simulink model "rec_i2s"  (R2023b)
settings: Solver=VariableStepAuto  StartTime=0.0  StopTime=10  RelTol=1e-3
values from neighbouring files (symbols this model uses):
  cnt1_LRCLK = 511    [DATA_GEN.m]
  cnt2_SCLK = 7    [DATA_GEN.m]
libraries: hdlsllib x3, eeGeneralControl x1
settings Model: Creator=31651  LastModifiedBy=31651
settings OptimizationCC: BlockReduction=off  ConditionallyExecuteInputs=off

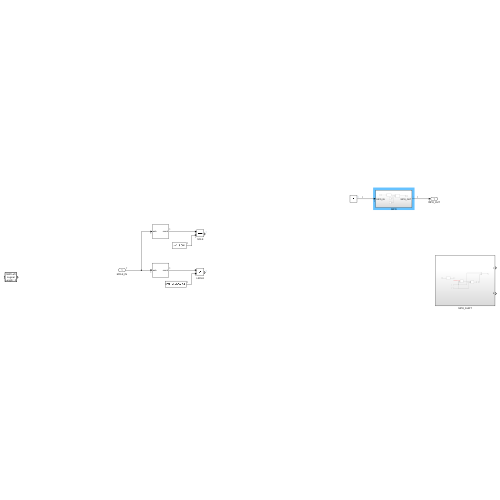
[thumbnail: Simulink's stored preview of the top-level diagram]
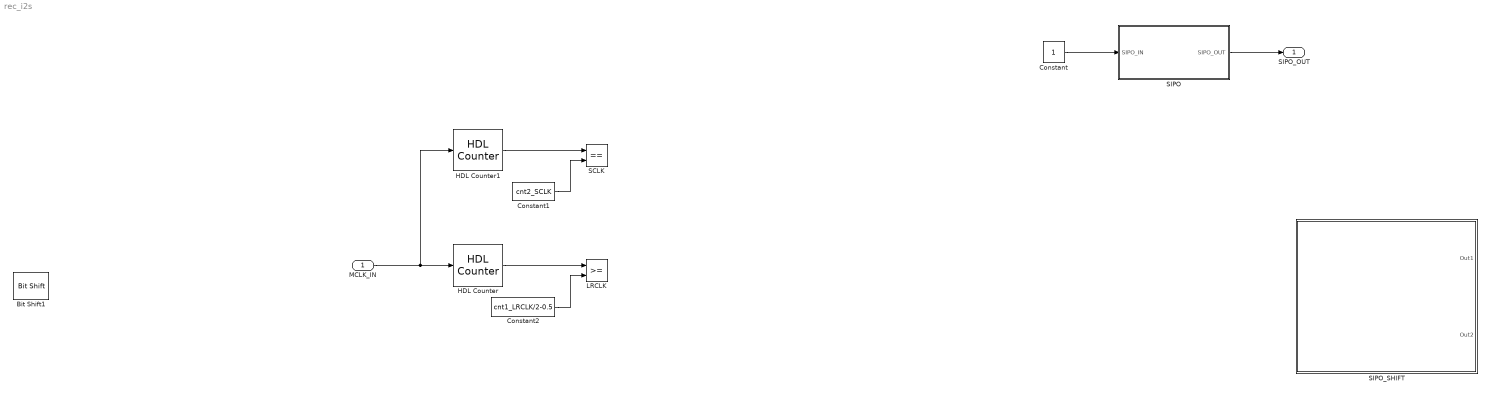
== system rec_i2s ==
  MCLK_IN : Inport
  Bit Shift1 : hdlsllib/Logic and Bit Operations/Bit Shift  mode=Shift Left Logical  N=0
  Constant : Constant  OutDataTypeStr=boolean  SampleTime=1
  Constant1 : Constant  Value=cnt2_SCLK  OutDataTypeStr=uint16
  Constant2 : Constant  Value=cnt1_LRCLK/2-0.5  OutDataTypeStr=uint16
  HDL Counter : hdlsllib/Sources/HDL Counter  CountType=Count limited  CountInit=0  CountStep=1  CountMax=cnt1_LRCLK  CountFromType=Initial value  CountFrom=0  CountResetPort=off  CountLoadPort=off  CountEnbPort=on  CountDirPort=off  CountHitOutputPort=off  CountDataType=Unsigned  CountWordLen=16  CountFracLen=0  CountSampTime=1
  HDL Counter1 : hdlsllib/Sources/HDL Counter  CountType=Count limited  CountInit=0  CountStep=1  CountMax=cnt2_SCLK  CountFromType=Initial value  CountFrom=0  CountResetPort=off  CountLoadPort=off  CountEnbPort=on  CountDirPort=off  CountHitOutputPort=off  CountDataType=Unsigned  CountWordLen=16  CountFracLen=0  CountSampTime=1
  LRCLK : RelationalOperator  OutDataTypeStr=boolean  InputSameDT=off
  SCLK : RelationalOperator  Operator===  OutDataTypeStr=boolean  InputSameDT=off
  SIPO : Subsystem
  SIPO_SHIFT : Subsystem
  SIPO_OUT : Outport  VectorParamsAs1DForOutWhenUnconnected=off
  wires:
  Constant1/1 -> SCLK/2
  HDL Counter1/1 -> SCLK/1
  Constant2/1 -> LRCLK/2
  MCLK_IN/1 -> HDL Counter/1, HDL Counter1/1
  HDL Counter/1 -> LRCLK/1
  Constant/1 -> SIPO/1(SIPO_IN)
  SIPO/1(SIPO_OUT) -> SIPO_OUT/1

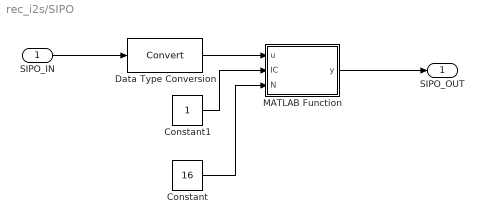
== system rec_i2s/SIPO ==
  SIPO_IN : Inport
  Constant : Constant  Value=16  SampleTime=1
  Constant1 : Constant  SampleTime=1
  Data Type Conversion : DataTypeConversion  SaturateOnIntegerOverflow=off  RndMeth=Floor
  MATLAB Function : MATLAB Function  TreatAsAtomicUnit=on
  SIPO_OUT : Outport  VectorParamsAs1DForOutWhenUnconnected=off
  wires:
  Data Type Conversion/1 -> MATLAB Function/1(u)
  MATLAB Function/1(y) -> SIPO_OUT/1
  SIPO_IN/1 -> Data Type Conversion/1
  Constant/1 -> MATLAB Function/3(N)
  Constant1/1 -> MATLAB Function/2(IC)

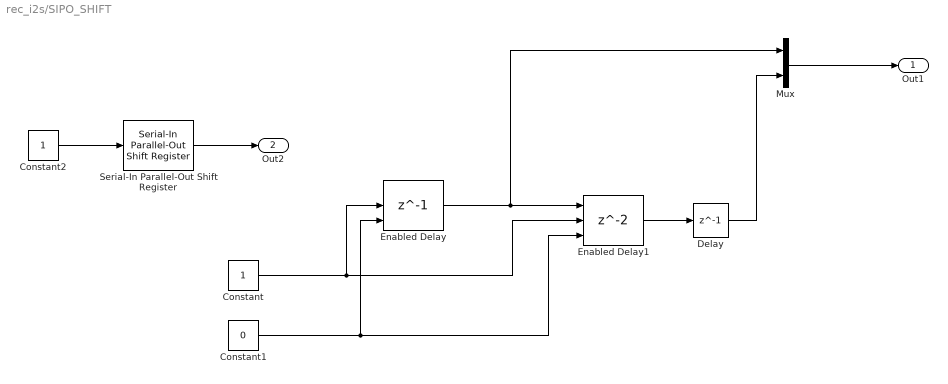
== system rec_i2s/SIPO_SHIFT ==
  Constant : Constant  OutDataTypeStr=boolean  SampleTime=1
  Constant1 : Constant  Value=0  OutDataTypeStr=boolean  SampleTime=1
  Constant2 : Constant  OutDataTypeStr=boolean  SampleTime=1
  Delay : Delay  DelayLength=1  InitialCondition=0
  Enabled Delay : Delay  DelayLength=1  ExternalReset=Level  ShowEnablePort=on
      settings: InputPortMap=u0,e6,r5
  Enabled Delay1 : Delay  ExternalReset=Level  ShowEnablePort=on
      settings: InputPortMap=u0,e6,r5
  Mux : Mux  Inputs=2
  Serial-In Parallel-Out Shift Register : eeGeneralControl/Serial-In Parallel-Out Shift Register  N=10  IC=0  Ts=-1
      settings: LibrarySourceBlock=|
      | ee_sl_lib/General Control/Serial-In Parallel-Out
      | Shift Register
  Out1 : Outport  VectorParamsAs1DForOutWhenUnconnected=off
  Out2 : Outport  Port=2  VectorParamsAs1DForOutWhenUnconnected=off
  wires:
  Enabled Delay/1 -> Mux/1, Enabled Delay1/1
  Constant/1 -> Enabled Delay/2, Enabled Delay1/2
  Enabled Delay1/1 -> Delay/1
  Delay/1 -> Mux/2
  Mux/1 -> Out1/1
  Constant1/1 -> Enabled Delay/3, Enabled Delay1/3
  ? -> Enabled Delay/1
  Constant2/1 -> Serial-In Parallel-Out Shift Register/1
  Serial-In Parallel-Out Shift Register/1 -> Out2/1

== matlab function rec_i2s/SIPO/MATLAB Function ==
  data: u input; y output; IC input; N input
function y = fcn(u,IC, N)
%#codegen

persistent buffer;

if isempty(buffer)
    buffer = IC*ones(N,length(u));
end

% Update buffer
buffer = [u'; buffer(1:end-1,:)];

% Update output
y = reshape(buffer,length(u)*N,1);

end
